simulink model "seminar6_2"  (R2015b)
settings: Solver=ode4  StartTime=0.0  StopTime=10  FixedStep=1e-6  RelTol=1e-3
libraries: powerlib x12, simulink x1
settings Model: Creator=Administrator  LastModifiedBy=Administrator

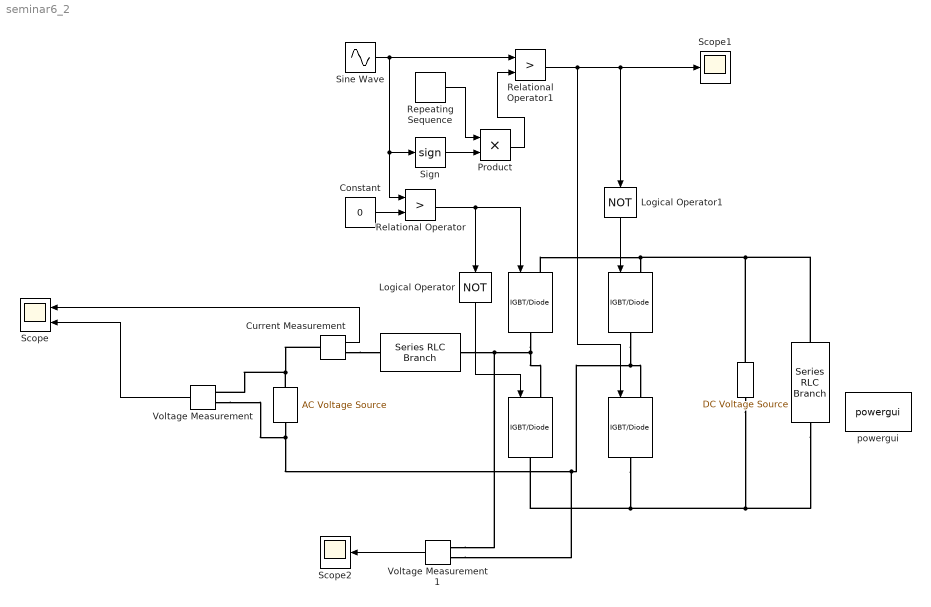
== system seminar6_2 ==
   {,,,} (4 alike) : powerlib/Power Electronics/IGBT//Diode  Ron=1e-3  Rs=1e5  Cs=inf  Measurements=off
  " " : powerlib/Electrical Sources/AC Voltage Source  Amplitude=311  Phase=0  Frequency=50  SampleTime=0  Measurements=None  BusType=swing  Pref=10e3  Qref=0  Qmin=-inf  Qmax=+inf
  " " : powerlib/Elements/Series RLC Branch  LConnTagsString=__new0  RConnTagsString=__new0  BranchType=L  Resistance=1  Inductance=4e-3  SetiL0=off  InitialCurrent=0  Capacitance=1e-6  Setx0=off  InitialVoltage=0  Measurements=None
  " " : powerlib/Electrical Sources/DC Voltage Source  Amplitude=550  Measurements=None
  " " : powerlib/Elements/Series RLC Branch  LConnTagsString=__new0  RConnTagsString=__new0  BranchType=R  Resistance=1  Inductance=1e-3  SetiL0=off  InitialCurrent=0  Capacitance=1e-6  Setx0=off  InitialVoltage=0  Measurements=None
  Constant : Constant  Value=0
  Current Measurement : powerlib/Measurements/Current Measurement  PhasorSimulation=off  OutputType=Complex  PSBequivalent=0
  Logical Operator : Logic  Operator=NOT  AllPortsSameDT=off  OutDataTypeStr=boolean
  Logical Operator1 : Logic  Operator=NOT  AllPortsSameDT=off  OutDataTypeStr=boolean
  Product : Product
  Relational Operator : RelationalOperator  Operator=>  OutDataTypeStr=boolean
  Relational Operator1 : RelationalOperator  Operator=>  OutDataTypeStr=boolean
  Repeating Sequence : simulink/Sources/Repeating Sequence  rep_seq_t=[0 2.5e-5 5e-5]  rep_seq_y=[0 1 0]
  Scope : Scope  NumInputPorts=2
  Scope1 : Scope
  Scope2 : Scope
  Sign : Signum
  Sine Wave : Sin  Amplitude=0.53  Frequency=100*pi  Phase=-7.582*pi/180  SampleTime=0
  Voltage Measurement : powerlib/Measurements/Voltage Measurement  PhasorSimulation=off  OutputType=Complex  PSBequivalent=0
  Voltage Measurement1 : powerlib/Measurements/Voltage Measurement  PhasorSimulation=off  OutputType=Complex  PSBequivalent=0
  powergui : powerlib/powergui  Priority=1  SimulationMode=Continuous  SolverType=Tustin/Backward Euler (TBE)  SampleTime=50e-6  frequency=60  SPID=off  DisableSnubberDevices=off  DisableRonSwitches=off  DisableVfSwitches=off  SwTol=0  DisplayEquations=off  Interpol=off  ExternalGateDelay=off  methode=off  Ts=10  FunctionMessages=off  echomessages=off  HookPort=off  EnableUseOfTLC=off  x0status=blocks  frequencyindice=0  Pbase=100e6  ErrMax=1e-4  Iterations=50  UnitsV=kV  UnitsW=MW  buscounter=0  RestoreLinks=warning  ResistiveCurrentMeasurement=off  Frange=[0:2:500]  Ylog=off  Xlog=on  ShowGrid=off  save=off  variable=ZData  structure=Uab  ZoomFFT=off  StartTime=0  cycles=2  DisplayStyle=2  fundamental=50  FreqAxis=off  MaxFrequency=1000  frequencyindicesteady=1  RmsSteady=1  display=off
  wires:
  Constant/1 -> Relational Operator/2
  Sine Wave/1 -> Relational Operator1/1, Sign/1, Relational Operator/1
  Relational Operator/1 -> " "/1, Logical Operator/1
  Logical Operator/1 -> " "/1
  Repeating Sequence/1 -> Product/1
  Relational Operator1/1 -> " "/1, Logical Operator1/1, Scope1/1
  Logical Operator1/1 -> " "/1
  Voltage Measurement/1 -> Scope/2
  Sign/1 -> Product/2
  Product/1 -> Relational Operator1/2
  Voltage Measurement1/1 -> Scope2/1
  Current Measurement/1 -> Scope/1
  connections:
  " "/RConn1 -- Current Measurement/LConn1 -- Voltage Measurement/LConn1
  " "/RConn1 -- Voltage Measurement1/LConn1 -- " "/LConn1
  " "/RConn1 -- Voltage Measurement1/LConn2 -- Voltage Measurement/LConn2 -- " "/LConn1
  " "/LConn1 -- " "/RConn1
  " "/LConn1 -- " "/RConn1
  Current Measurement/RConn1 -- " "/LConn1
